simulink model "Scenario_MinimumExample_TwithTrafficLights_tol_fixed"  (R2021a)
settings: Solver=VariableStepAuto  StartTime=0.0  StopTime=50  RelTol=1e-3
model workspace (MAT data in the model file):
  Kz_dif = Simulink.Parameter
  Kz_dif.Value = Simulink.data.Expression
  Kz_dif.Value.ExpressionString = " L_dif / (Lc + ds)"
  Kz_dif.DataType = 'auto'
  Kz_dif.Dimensions = -1
  Kz_il = Simulink.Parameter
  Kz_il.Value = Simulink.data.Expression
  Kz_il.Value.ExpressionString = " L_il / (Lc + ds)"
  Kz_il.DataType = 'auto'
  Kz_il.Dimensions = -1
  Kz_ir = Simulink.Parameter
  Kz_ir.Value = Simulink.data.Expression
  Kz_ir.Value.ExpressionString = " L_ir / (Lc + ds)"
  Kz_ir.DataType = 'auto'
  Kz_ir.Dimensions = -1
  Kz_is = Simulink.Parameter
  Kz_is.Value = Simulink.data.Expression
  Kz_is.Value.ExpressionString = " L_is / (Lc + ds)"
  Kz_is.DataType = 'auto'
  Kz_is.Dimensions = -1
  Kz_long = Simulink.Parameter
  Kz_long.Value = Simulink.data.Expression
  Kz_long.Value.ExpressionString = " L_long / (Lc + ds)"
  Kz_long.Description = 'Segmentkapazität (wie viele autos passen hinein)'
  Kz_long.DataType = 'auto'
  Kz_long.Dimensions = -1
  Kz_pre = Simulink.Parameter
  Kz_pre.Value = Simulink.data.Expression
  Kz_pre.Value.ExpressionString = " L_pre / (Lc + ds)"
  Kz_pre.DataType = 'auto'
  Kz_pre.Dimensions = -1
  L_dif = Simulink.Parameter
  L_dif.Value = Simulink.data.Expression
  L_dif.Value.ExpressionString = "L_long-L_pre"
  L_dif.Description = 'Differenz zwischen Abbiegerspurlänge und normaler straßenlänge'
  L_dif.DataType = 'auto'
  L_dif.Dimensions = -1
  L_il = Simulink.Parameter
  L_il.Value = 30
  L_il.Description = 'Länge der innenkreuzungssegments, das linksabbieger durchqueren'
  L_il.DataType = 'auto'
  L_il.Dimensions = [1 1]
  L_ir = Simulink.Parameter
  L_ir.Value = 23
  L_ir.Description = 'Länge der innenkreuzungssegments, das rechtsabbieger durchqueren'
  L_ir.DataType = 'auto'
  L_ir.Dimensions = [1 1]
  L_is = Simulink.Parameter
  L_is.Value = 35
  L_is.Description = 'Länge der innenkreuzungssegments, das geradeausfahrer durchqueren'
  L_is.DataType = 'auto'
  L_is.Dimensions = [1 1]
  L_long = Simulink.Parameter
  L_long.Value = 52.8
  L_long.Description = 'Langes straßensegment  (52.8 meter)'
  L_long.DataType = 'auto'
  L_long.Dimensions = [1 1]
  L_pre = Simulink.Parameter
  L_pre.Value = 20
  L_pre.Description = 'Länge der Abbiegespuren'
  L_pre.DataType = 'auto'
  L_pre.Dimensions = [1 1]
  Lc = Simulink.Parameter
  Lc.Value = 4.4
  Lc.Description = 'Länge eines autos'
  Lc.DataType = 'auto'
  Lc.Dimensions = [1 1]
  Rk = Simulink.Parameter
  Rk.Value = Simulink.data.Expression
  Rk.Value.ExpressionString = " 1 / (Lc / v)"
  Rk.Description = 'Flussrate zwischen den Kanten (bei speed v)'
  Rk.DataType = 'auto'
  Rk.Dimensions = -1
  Tz_dif = Simulink.Parameter
  Tz_dif.Value = Simulink.data.Expression
  Tz_dif.Value.ExpressionString = " L_dif / v"
  Tz_dif.DataType = 'auto'
  Tz_dif.Dimensions = -1
  Tz_il = Simulink.Parameter
  Tz_il.Value = Simulink.data.Expression
  Tz_il.Value.ExpressionString = " L_il / v"
  Tz_il.DataType = 'auto'
  Tz_il.Dimensions = -1
  Tz_ir = Simulink.Parameter
  Tz_ir.Value = Simulink.data.Expression
  Tz_ir.Value.ExpressionString = " L_ir / v"
  Tz_ir.DataType = 'auto'
  Tz_ir.Dimensions = -1
  Tz_is = Simulink.Parameter
  Tz_is.Value = Simulink.data.Expression
  Tz_is.Value.ExpressionString = " L_is / v"
  Tz_is.DataType = 'auto'
  Tz_is.Dimensions = -1
  Tz_long = Simulink.Parameter
  Tz_long.Value = Simulink.data.Expression
  Tz_long.Value.ExpressionString = " L_long / v"
  Tz_long.Description = 'Segment durchfahrtzeit: wie lange würde ein auto brauchen,um
    | ungehindert durch das segment zu fahren.'
  Tz_long.DataType = 'auto'
  Tz_long.Dimensions = -1
  Tz_pre = Simulink.Parameter
  Tz_pre.Value = Simulink.data.Expression
  Tz_pre.Value.ExpressionString = " L_pre / v"
  Tz_pre.DataType = 'auto'
  Tz_pre.Dimensions = -1
  ds = Simulink.Parameter
  ds.Value = Simulink.data.Expression
  ds.Value.ExpressionString = "v*dt"
  ds.DataType = 'auto'
  ds.Dimensions = -1
  dt = Simulink.Parameter
  dt.Value = 1
  dt.Description = 'temporaler sicherheitsabstand'
  dt.DataType = 'auto'
  dt.Dimensions = [1 1]
  v = Simulink.Parameter
  v.Value = 13.89
  v.Description = 'geschwindigkeit eines autos
    | (km/h : 3.75 = m/s)
    | 	30km/h = 8,34m/s
    | 	20km/h = 5.56m/s
    | 	50km/h = 13.89m/s
    | '
  v.DataType = 'auto'
  v.Dimensions = [1 1]
libraries: StreetLanesLibrary x72, EdgesLibrary x64, MeasuringLibrary x33, SourcesAndSinksLibrary x12, LightsLibrary x2
(part 1 of 2)
settings Model: Creator=phill  LastModifiedBy=phill
settings SolverCC: ZeroCrossAlgorithm=Adaptive
settings DebuggingCC: IgnoredZcDiagnostic=none

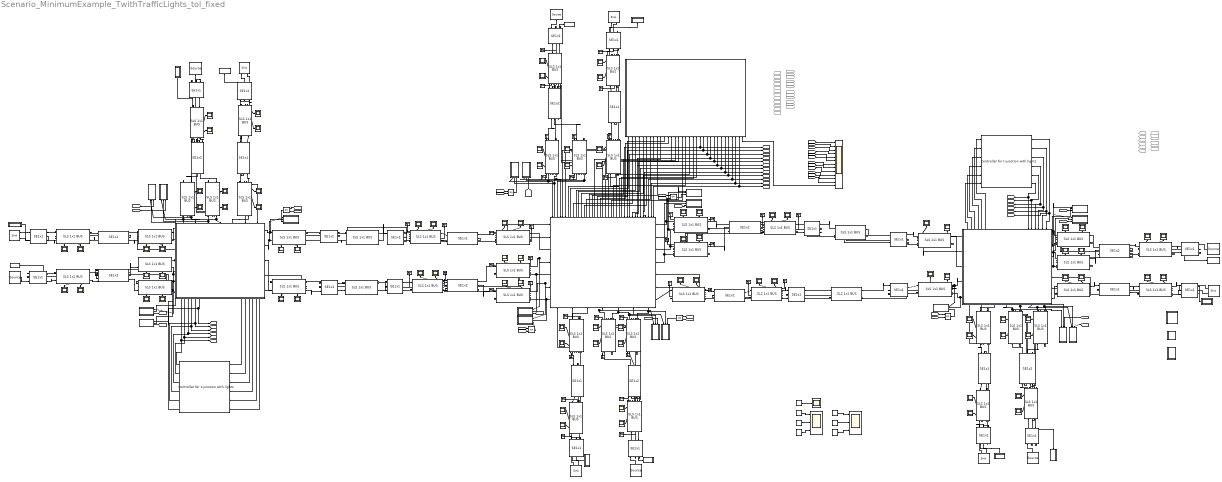
== system Scenario_MinimumExample_TwithTrafficLights_tol_fixed ==
  Ain : StreetLanesLibrary/SLS 1x1 BUS  Kz=Kz_dif  Tz=Tz_dif
  Ain2 : StreetLanesLibrary/SLS 1x1 BUS  Kz=Kz_dif  Tz=Tz_dif
  Ain3 : StreetLanesLibrary/SLS 1x1 BUS  Kz=Kz_dif  Tz=Tz_dif
  AinSplit : EdgesLibrary/SE1x2  Rk1=0.5*Rk  Rk2=0.5*Rk
  AinSplit2 : EdgesLibrary/SE1x2  Rk1=0.5*Rk  Rk2=0.5*Rk
  AinSplit3 : EdgesLibrary/SE1x2  Rk1=0.5*Rk  Rk2=0.5*Rk
  AinX : Scope
  AinX2 : Scope
  AinX3 : Scope
  AinY : Scope
  AinY2 : Scope
  AinY3 : Scope
  Al : StreetLanesLibrary/SLS 1x1 BUS  Kz=Kz_pre  Tz=Tz_pre
  AlX : Scope
  AlY : Scope
  Ali1 : StreetLanesLibrary/SLS 1x1 BUS  Kz=Kz_pre  Tz=Tz_pre
  Ali2 : StreetLanesLibrary/SLS 1x1 BUS  Kz=Kz_pre  Tz=Tz_pre
  AliX1 : Scope
  AliX2 : Scope
  AliY1 : Scope
  AliY2 : Scope
  Ao : StreetLanesLibrary/SLS 1x1 BUS  Kz=Kz_pre  Tz=Tz_pre
  Ao2 : StreetLanesLibrary/SLS 1x1 BUS  Kz=Kz_pre  Tz=Tz_pre
  Ao3 : StreetLanesLibrary/SLS 1x1 BUS  Kz=Kz_pre  Tz=Tz_pre
  AoX : Scope
  AoX2 : Scope
  AoX3 : Scope
  AoY : Scope
  AoY2 : Scope
  AoY3 : Scope
  Aout : StreetLanesLibrary/SLS 1x1 BUS  Kz=Kz_dif  Tz=Tz_dif
  Aout2 : StreetLanesLibrary/SLS 1x1 BUS  Kz=Kz_dif  Tz=Tz_dif
  Aout3 : StreetLanesLibrary/SLS 1x1 BUS  Kz=Kz_dif  Tz=Tz_dif
  AoutX : Scope
  AoutX2 : Scope
  AoutX3 : Scope
  AoutY : Scope
  AoutY2 : Scope
  AoutY3 : Scope
  Ari1 : StreetLanesLibrary/SLS 1x1 BUS  Kz=Kz_pre  Tz=Tz_pre
  Ari2 : StreetLanesLibrary/SLS 1x1 BUS  Kz=Kz_pre  Tz=Tz_pre
  AriX1 : Scope
  AriX2 : Scope
  AriY1 : Scope
  AriY2 : Scope
  Ars : StreetLanesLibrary/SLS 1x1 BUS  Kz=Kz_pre  Tz=Tz_pre
  ArsX : Scope
  ArsY : Scope
  Bin : StreetLanesLibrary/SLS 1x1 BUS  Kz=Kz_dif  Tz=Tz_dif
  BinSplit1 : EdgesLibrary/SE1x2  Rk1=0.5*Rk  Rk2=0.5*Rk
  BinX : Scope
  BinY : Scope
  Bl : StreetLanesLibrary/SLS 1x1 BUS  Kz=Kz_pre  Tz=Tz_pre
  BlX : Scope
  BlY : Scope
  Bo : StreetLanesLibrary/SLS 1x1 BUS  Kz=Kz_pre  Tz=Tz_pre
  Bo2 : StreetLanesLibrary/SLS 1x1 BUS  Kz=Kz_pre  Tz=Tz_pre
  Bo3 : StreetLanesLibrary/SLS 1x1 BUS  Kz=Kz_long  Tz=Tz_long
  Bo4 : StreetLanesLibrary/SLS 1x1 BUS  Kz=Kz_pre  Tz=Tz_pre
  BoX : Scope
  BoX2 : Scope
  BoX3 : Scope
  BoY : Scope
  BoY2 : Scope
  BoY3 : Scope
  Bout : StreetLanesLibrary/SLS 1x1 BUS  Kz=Kz_dif  Tz=Tz_dif
  BoutX : Scope
  BoutY : Scope
  Brs : StreetLanesLibrary/SLS 1x1 BUS  Kz=Kz_pre  Tz=Tz_pre
  Brs2 : StreetLanesLibrary/SLS 1x1 BUS  Kz=Kz_pre  Tz=Tz_pre
  Brs3 : StreetLanesLibrary/SLS 1x1 BUS  Kz=Kz_long  Tz=Tz_long
  Brs4 : StreetLanesLibrary/SLS 1x1 BUS  Kz=Kz_pre  Tz=Tz_pre
  BrsX : Scope
  BrsX2 : Scope
  BrsX3 : Scope
  BrsY : Scope
  BrsY2 : Scope
  BrsY3 : Scope
  Cin : StreetLanesLibrary/SLS 1x1 BUS  Kz=Kz_dif  Tz=Tz_dif
  Cin2 : StreetLanesLibrary/SLS 1x1 BUS  Kz=Kz_dif  Tz=Tz_dif
  Cin3 : StreetLanesLibrary/SLS 1x1 BUS  Kz=Kz_long  Tz=Tz_long
  Cin4 : StreetLanesLibrary/SLS 1x1 BUS  Kz=Kz_dif  Tz=Tz_dif
  CinSplit : EdgesLibrary/SE1x2  Rk1=0.5*Rk  Rk2=0.5*Rk
  CinSplit2 : EdgesLibrary/SE1x2  Rk1=0.5*Rk  Rk2=0.5*Rk
  CinSplit3 : EdgesLibrary/SE1x2  Rk1=0.5*Rk  Rk2=0.5*Rk
  CinX : Scope
  CinX2 : Scope
  CinX3 : Scope
  CinY : Scope
  CinY2 : Scope
  CinY3 : Scope
  Cl : StreetLanesLibrary/SLS 1x1 BUS  Kz=Kz_pre  Tz=Tz_pre
  Cl2 : StreetLanesLibrary/SLS 1x1 BUS  Kz=Kz_pre  Tz=Tz_pre
  Cl3 : StreetLanesLibrary/SLS 1x1 BUS  Kz=Kz_pre  Tz=Tz_pre
  ClX : Scope
  ClX2 : Scope
  ClX3 : Scope
  ClY1 : Scope
  ClY2 : Scope
  Cly : Scope
  Co : StreetLanesLibrary/SLS 1x1 BUS  Kz=Kz_pre  Tz=Tz_pre
  Co2 : StreetLanesLibrary/SLS 1x1 BUS  Kz=Kz_pre  Tz=Tz_pre
  Co3 : StreetLanesLibrary/SLS 1x1 BUS  Kz=Kz_pre  Tz=Tz_pre
  CoX : Scope
  CoX2 : Scope
  CoX3 : Scope
  CoY : Scope
  CoY2 : Scope
  CoY3 : Scope
  Controller for t-junction with lights : LightsLibrary/Controller for t-junction with lights  green_time=5
  Controller for t-junction with lights1 : LightsLibrary/Controller for t-junction with lights  green_time=5
  Cout{,2..4} (4 alike) : StreetLanesLibrary/SLS 1x1 BUS  Kz=Kz_dif  Tz=Tz_dif
  CoutX : Scope
  CoutX2 : Scope
  CoutX3 : Scope
  CoutY : Scope
  CoutY2 : Scope
  CoutY3 : Scope
  Crs : StreetLanesLibrary/SLS 1x1 BUS  Kz=Kz_pre  Tz=Tz_pre
  CrsX : Scope
  CrsY : Scope
  Cs1 : StreetLanesLibrary/SLS 1x1 BUS  Kz=Kz_pre  Tz=Tz_pre
  Cs2 : StreetLanesLibrary/SLS 1x1 BUS  Kz=Kz_pre  Tz=Tz_pre
  CsX1 : Scope
  CsX2 : Scope
  CsY1 : Scope
  CsY2 : Scope
  Din : StreetLanesLibrary/SLS 1x1 BUS  Kz=Kz_dif  Tz=Tz_dif
  DinSplit : EdgesLibrary/SE1x2  Rk1=0.5*Rk  Rk2=0.5*Rk
  DinX : Scope
  DinY : Scope
  Dl : StreetLanesLibrary/SLS 1x1 BUS  Kz=Kz_pre  Tz=Tz_pre
  DlX : Scope
  DlY : Scope
  Do : StreetLanesLibrary/SLS 1x1 BUS  Kz=Kz_pre  Tz=Tz_pre
  DoX : Scope
  DoY : Scope
  Dout : StreetLanesLibrary/SLS 1x1 BUS  Kz=Kz_dif  Tz=Tz_dif
  DoutX : Scope
  DoutY : Scope
  Drs : StreetLanesLibrary/SLS 1x1 BUS  Kz=Kz_pre  Tz=Tz_pre
  DrsX : Scope
  DrsY : Scope
  From24 : From  Commented=on  GotoTag=CenAl
  From25 : From  Commented=on  GotoTag=CenAs
  From26 : From  Commented=on  GotoTag=CenDs
  From27 : From  Commented=on  GotoTag=CenDr
  From28 : From  Commented=on  GotoTag=CenAr
  From29 : From  Commented=on  GotoTag=CenBl
  From30 : From  Commented=on  GotoTag=CenBs
  From31 : From  Commented=on  GotoTag=CenBr
  From32 : From  Commented=on  GotoTag=CenCl
  From33 : From  Commented=on  GotoTag=CenCs
  From34 : From  Commented=on  GotoTag=CenCr
  From35 : From  Commented=on  GotoTag=CenDl
  From42 : From  Commented=on  GotoTag=RenCs
  From43 : From  Commented=on  GotoTag=RenCl
  From44 : From  Commented=on  GotoTag=RenAr
  From45 : From  Commented=on  GotoTag=RenAl
  From46 : From  Commented=on  GotoTag=RenBr
  From47 : From  Commented=on  GotoTag=RenBs
  Goto24 : Goto  Commented=on  GotoTag=CenAl
  Goto25 : Goto  Commented=on  GotoTag=CenAs
  Goto26 : Goto  Commented=on  GotoTag=CenDs
  Goto27 : Goto  Commented=on  GotoTag=CenDr
  Goto28 : Goto  Commented=on  GotoTag=CenAr
  Goto29 : Goto  Commented=on  GotoTag=CenBl
  Goto30 : Goto  Commented=on  GotoTag=CenBs
  Goto31 : Goto  Commented=on  GotoTag=CenBr
  Goto32 : Goto  Commented=on  GotoTag=CenCl
  Goto33 : Goto  Commented=on  GotoTag=CenCs
  Goto34 : Goto  Commented=on  GotoTag=CenCr
  Goto35 : Goto  Commented=on  GotoTag=CenDl
  Goto42 : Goto  Commented=on  GotoTag=RenCl
  Goto43 : Goto  Commented=on  GotoTag=RenCs
  Goto44 : Goto  Commented=on  GotoTag=RenBs
  Goto45 : Goto  Commented=on  GotoTag=RenBr
  Goto46 : Goto  Commented=on  GotoTag=RenAl
  Goto47 : Goto  Commented=on  GotoTag=RenAr
  Kz_dif : Constant  Value=Kz_dif
  Kz_long : Constant  Value=Kz_long
  Kz_pre : Constant  Value=Kz_pre
  Kzs : Scope  NumInputPorts=3
  Logical Operator{,1..5} (6 alike) : Logic  Operator=OR  AllPortsSameDT=off  OutDataTypeStr=boolean
  Plus-Controller : Stateflow chart  TreatAsAtomicUnit=on  mask{green_duration_sr=6, green_duration_l=6, tol=0}
      mask prompts: green_duration_sr "Green Duration for straight/right traffic"; green_duration_l "Green Duration for left traffic"; tol "tolerance"
      settings: PortSchema="{\"entries\":[{\"content\":{\"sides\":[{\"content\":{\"connectorIds\":[]},\"type\":\"ConnectorPlacement.EquallySpacedRectSide\",\"uuid\":\"2590cc03-86a2-4387-8b1b-fdf4c8b68aa6\"},{\"content\":{\"connectorIds\":[],\"side\":\"RIGHT\"},\"type\":\"ConnectorPlacement.EquallySpacedRectSide\",\"uuid\":\"b97063cd-dd31-425f-b4aa-3aaa013ac411\"},{\"content\":{\"connectorIds\":[],\"side\":\"TOP\"},\"type\":\"ConnectorPlacement.EquallySpacedRectSide\",\"uuid\":\"ef5846b9-436e-4b10-a854-1305521b6a0d\"},{\"content\":{\"connectorIds\":[\"In3\",\"In4\",\"In1\",\"In2\",\"In5\",\"In6\",\"In7\",\"In8\",\"In9\",\"In10\",\"In11\",\"In12\",\"In13\",\"In14\",\"In15\",\"In16\",\"In17\",\"In18\",\"In19\",\"In20\",\"Out1\",\"Out2\",\"Out3\",\"Out4\",\"Out5\",\"Out6\",\"Out7\",\"Out8\",\"Out9\",\"Out10\",\"Out11\",\"Out12\",\"Out13\"],\"side\":\"BOTTOM\"},\"type\":\"ConnectorPlacement.EquallySpacedRectSide\",\"uuid\":\"44b73820-3b7c-4ee5-b5da-9465e85a924e\"}]},\"type\":\"ConnectorPlacement.EquallySpacedConnector\",\"uuid\":\"3342797d-7762-4a2a-891a-654024402a66\"}],\"packageUris\":[\"http://schema.mathworks.com/mf0/Connector/R2020b\"],\"version\":\"1.0\"}"
  Rk : Constant  Value=Rk
  SE1x{1..4,7..10} (8 alike) : EdgesLibrary/SE1x1  Rk=Rk  slope=2000
  Scope : Scope  NumInputPorts=13
  Sink A : SourcesAndSinksLibrary/Sink  SystemSampleTime=-1  VariantActivationTime=update diagram  Latency=0  AutoFrameSizeCalculation=off
      settings: PortSchema="{\"entries\":[{\"content\":{\"sides\":[{\"content\":{\"connectorIds\":[\"Out1\",\"Out2\"]},\"type\":\"ConnectorPlacement.EquallySpacedRectSide\",\"uuid\":\"9fd2383e-3590-4f0f-bafc-5a4adfbb32b4\"},{\"content\":{\"connectorIds\":[],\"side\":\"RIGHT\"},\"type\":\"ConnectorPlacement.EquallySpacedRectSide\",\"uuid\":\"1e687aa9-1098-45bd-a1f6-ea403f3f2897\"},{\"content\":{\"connectorIds\":[],\"side\":\"TOP\"},\"type\":\"ConnectorPlacement.EquallySpacedRectSide\",\"uuid\":\"fe6eaa71-085c-414b-983a-a0e72e52a49c\"}]},\"type\":\"ConnectorPlacement.EquallySpacedConnector\",\"uuid\":\"370c1712-4373-4726-99c2-6cb04807ece1\"}],\"packageUris\":[\"http://schema.mathworks.com/mf0/Connector/R2020b\"],\"version\":\"1.0\"}"
  Sink A2 : SourcesAndSinksLibrary/Sink  SystemSampleTime=-1  VariantActivationTime=update diagram  Latency=0  AutoFrameSizeCalculation=off
      settings: PortSchema="{\"entries\":[{\"content\":{\"sides\":[{\"content\":{\"connectorIds\":[\"Out1\",\"Out2\"]},\"type\":\"ConnectorPlacement.EquallySpacedRectSide\",\"uuid\":\"9fd2383e-3590-4f0f-bafc-5a4adfbb32b4\"},{\"content\":{\"connectorIds\":[],\"side\":\"RIGHT\"},\"type\":\"ConnectorPlacement.EquallySpacedRectSide\",\"uuid\":\"1e687aa9-1098-45bd-a1f6-ea403f3f2897\"},{\"content\":{\"connectorIds\":[],\"side\":\"TOP\"},\"type\":\"ConnectorPlacement.EquallySpacedRectSide\",\"uuid\":\"fe6eaa71-085c-414b-983a-a0e72e52a49c\"}]},\"type\":\"ConnectorPlacement.EquallySpacedConnector\",\"uuid\":\"370c1712-4373-4726-99c2-6cb04807ece1\"}],\"packageUris\":[\"http://schema.mathworks.com/mf0/Connector/R2020b\"],\"version\":\"1.0\"}"
  Sink A3 : SourcesAndSinksLibrary/Sink  SystemSampleTime=-1  VariantActivationTime=update diagram  Latency=0  AutoFrameSizeCalculation=off
      settings: PortSchema="{\"entries\":[{\"content\":{\"sides\":[{\"content\":{\"connectorIds\":[\"Out1\",\"Out2\"]},\"type\":\"ConnectorPlacement.EquallySpacedRectSide\",\"uuid\":\"9fd2383e-3590-4f0f-bafc-5a4adfbb32b4\"},{\"content\":{\"connectorIds\":[],\"side\":\"RIGHT\"},\"type\":\"ConnectorPlacement.EquallySpacedRectSide\",\"uuid\":\"1e687aa9-1098-45bd-a1f6-ea403f3f2897\"},{\"content\":{\"connectorIds\":[],\"side\":\"TOP\"},\"type\":\"ConnectorPlacement.EquallySpacedRectSide\",\"uuid\":\"fe6eaa71-085c-414b-983a-a0e72e52a49c\"}]},\"type\":\"ConnectorPlacement.EquallySpacedConnector\",\"uuid\":\"370c1712-4373-4726-99c2-6cb04807ece1\"}],\"packageUris\":[\"http://schema.mathworks.com/mf0/Connector/R2020b\"],\"version\":\"1.0\"}"
  Sink C : SourcesAndSinksLibrary/Sink  SystemSampleTime=-1  VariantActivationTime=update diagram  Latency=0  AutoFrameSizeCalculation=off
      settings: PortSchema="{\"entries\":[{\"content\":{\"sides\":[{\"content\":{\"connectorIds\":[\"Out1\",\"Out2\"]},\"type\":\"ConnectorPlacement.EquallySpacedRectSide\",\"uuid\":\"9fd2383e-3590-4f0f-bafc-5a4adfbb32b4\"},{\"content\":{\"connectorIds\":[],\"side\":\"RIGHT\"},\"type\":\"ConnectorPlacement.EquallySpacedRectSide\",\"uuid\":\"1e687aa9-1098-45bd-a1f6-ea403f3f2897\"},{\"content\":{\"connectorIds\":[],\"side\":\"TOP\"},\"type\":\"ConnectorPlacement.EquallySpacedRectSide\",\"uuid\":\"fe6eaa71-085c-414b-983a-a0e72e52a49c\"}]},\"type\":\"ConnectorPlacement.EquallySpacedConnector\",\"uuid\":\"370c1712-4373-4726-99c2-6cb04807ece1\"}],\"packageUris\":[\"http://schema.mathworks.com/mf0/Connector/R2020b\"],\"version\":\"1.0\"}"
  Sink C2 : SourcesAndSinksLibrary/Sink  SystemSampleTime=-1  VariantActivationTime=update diagram  Latency=0  AutoFrameSizeCalculation=off
      settings: PortSchema="{\"entries\":[{\"content\":{\"sides\":[{\"content\":{\"connectorIds\":[\"Out1\",\"Out2\"]},\"type\":\"ConnectorPlacement.EquallySpacedRectSide\",\"uuid\":\"9fd2383e-3590-4f0f-bafc-5a4adfbb32b4\"},{\"content\":{\"connectorIds\":[],\"side\":\"RIGHT\"},\"type\":\"ConnectorPlacement.EquallySpacedRectSide\",\"uuid\":\"1e687aa9-1098-45bd-a1f6-ea403f3f2897\"},{\"content\":{\"connectorIds\":[],\"side\":\"TOP\"},\"type\":\"ConnectorPlacement.EquallySpacedRectSide\",\"uuid\":\"fe6eaa71-085c-414b-983a-a0e72e52a49c\"}]},\"type\":\"ConnectorPlacement.EquallySpacedConnector\",\"uuid\":\"370c1712-4373-4726-99c2-6cb04807ece1\"}],\"packageUris\":[\"http://schema.mathworks.com/mf0/Connector/R2020b\"],\"version\":\"1.0\"}"
  Sink D : SourcesAndSinksLibrary/Sink  SystemSampleTime=-1  VariantActivationTime=update diagram  Latency=0  AutoFrameSizeCalculation=off
      settings: PortSchema="{\"entries\":[{\"content\":{\"sides\":[{\"content\":{\"connectorIds\":[\"Out1\",\"Out2\"]},\"type\":\"ConnectorPlacement.EquallySpacedRectSide\",\"uuid\":\"9fd2383e-3590-4f0f-bafc-5a4adfbb32b4\"},{\"content\":{\"connectorIds\":[],\"side\":\"RIGHT\"},\"type\":\"ConnectorPlacement.EquallySpacedRectSide\",\"uuid\":\"1e687aa9-1098-45bd-a1f6-ea403f3f2897\"},{\"content\":{\"connectorIds\":[],\"side\":\"TOP\"},\"type\":\"ConnectorPlacement.EquallySpacedRectSide\",\"uuid\":\"fe6eaa71-085c-414b-983a-a0e72e52a49c\"}]},\"type\":\"ConnectorPlacement.EquallySpacedConnector\",\"uuid\":\"370c1712-4373-4726-99c2-6cb04807ece1\"}],\"packageUris\":[\"http://schema.mathworks.com/mf0/Connector/R2020b\"],\"version\":\"1.0\"}"
  Source A : SourcesAndSinksLibrary/Source  SystemSampleTime=-1  VariantActivationTime=update diagram  Latency=0  AutoFrameSizeCalculation=off
  Source A2 : SourcesAndSinksLibrary/Source  SystemSampleTime=-1  VariantActivationTime=update diagram  Latency=0  AutoFrameSizeCalculation=off
  Source A3 : SourcesAndSinksLibrary/Source  SystemSampleTime=-1  VariantActivationTime=update diagram  Latency=0  AutoFrameSizeCalculation=off
  Source C : SourcesAndSinksLibrary/Source  SystemSampleTime=-1  VariantActivationTime=update diagram  Latency=0  AutoFrameSizeCalculation=off
  Source C2 : SourcesAndSinksLibrary/Source  SystemSampleTime=-1  VariantActivationTime=update diagram  Latency=0  AutoFrameSizeCalculation=off
  Source D : SourcesAndSinksLibrary/Source  SystemSampleTime=-1  VariantActivationTime=update diagram  Latency=0  AutoFrameSizeCalculation=off
  Subsystem : Subsystem  mask{Kz_left=Kz_il, Tz_left=Tz_il, Kz_straight=Kz_is, Tz_straight=Tz_is, Kz_right=Kz_ir, Tz_right=Tz_ir, Rk=Rk}
      settings: PortSchema="{\"entries\":[{\"content\":{\"sides\":[{\"content\":{\"connectorIds\":[\"In1\",\"In2\",\"Out30\",\"In3\",\"Out31\",\"In4\",\"Out32\"]},\"type\":\"ConnectorPlacement.EquallySpacedRectSide\",\"uuid\":\"223afcc5-5490-41e2-b2c1-0ac31bdd31f0\"},{\"content\":{\"connectorIds\":[\"In25\",\"Out1\",\"In26\",\"Out2\",\"In27\",\"In28\",\"Out3\"],\"side\":\"RIGHT\"},\"type\":\"ConnectorPlacement.EquallySpacedRectSide\",\"uuid\":\"e803e5ea-345a-49fc-8782-ffb100729ba0\"},{\"content\":{\"connectorIds\":[\"In5\",\"Out7\",\"Out8\",\"In6\",\"In7\",\"In8\",\"Out9\",\"Out10\",\"Out11\",\"Out12\",\"Out13\",\"Out14\",\"Out15\",\"Out16\",\"Out17\",\"Out18\",\"Out19\",\"Out20\",\"Out21\",\"Out22\",\"Out23\",\"Out24\",\"Out25\",\"Out26\",\"Out27\",\"Out28\",\"Out29\",\"In9\",\"In10\",\"In11\",\"In12\",\"In13\",\"In14\",\"In15\",\"In16\",\"In17\",\"In18\",\"In19\",\"In20\"],\"side\":\"TOP\"},\"type\":\"ConnectorPlacement.EquallySpacedRectSide\",\"uuid\":\"8581fbf9-6742-4a7a-9e93-ed29b1a56c31\"},{\"content\":{\"connectorIds\":[\"In21\",\"In22\",\"Out4\",\"In23\",\"Out5\",\"In24\",\"Out6\"],\"side\":\"BOTTOM\"},\"type\":\"ConnectorPlacement.EquallySpacedRectSide\",\"uuid\":\"cc67de78-9dd9-463d-9445-caa2eb7c099b\"}]},\"type\":\"ConnectorPlacement.EquallySpacedConnector\",\"uuid\":\"ac6fc4cc-2326-4bcf-896c-a5d089a8f47a\"}],\"packageUris\":[\"http://schema.mathworks.com/mf0/Connector/R2020b\"],\"version\":\"1.0\"}"
      mask Display:
      | %image('$imagefile'); % Use "Edit Image" on toolstrip to change.
      | disp('+ \n\n');
      | KzS = get_param(gcb,'Kz_straight');
      | TzS = get_param(gcb,'Tz_straight');
      | KzR = get_param(gcb,'Kz_right');
      | TzR = get_param(gcb,'Tz_right');
      | KzL = get_param(gcb,'Kz_left');
      | TzL = get_param(gcb,'Tz_left');
      | Rk = get_param(gcb,'Rk');
      | disp(['Rk = ', Rk, ' | Kz/Tz L = ', KzL, ' ', TzL, ' | Kz/Tz S = ', KzS, ' ', TzS, ' | Kz/Tz R = ', KzR, ' ', TzR]);
  Subsystem1 : Subsystem  mask{Kz_left=Kz_il, Tz_left=Tz_il, Kz_straight=Kz_is, Tz_straight=Tz_is, Kz_right=Kz_ir, Tz_right=Tz_ir, Rk=Rk}
      settings: PortSchema="{\"entries\":[{\"content\":{\"sides\":[{\"content\":{\"connectorIds\":[\"In1\",\"In2\",\"Out24\",\"In3\",\"Out25\"]},\"type\":\"ConnectorPlacement.EquallySpacedRectSide\",\"uuid\":\"96c9f498-b0bc-4839-a476-8992d885d35a\"},{\"content\":{\"connectorIds\":[\"In14\",\"Out1\",\"In15\",\"Out2\",\"In16\",\"In17\",\"Out3\"],\"side\":\"RIGHT\"},\"type\":\"ConnectorPlacement.EquallySpacedRectSide\",\"uuid\":\"11ab0cdd-7db6-4f39-a252-8216aa6322d2\"},{\"content\":{\"connectorIds\":[\"Out7\",\"Out8\",\"Out9\",\"Out10\",\"Out11\",\"Out12\",\"Out13\",\"Out14\",\"Out15\",\"Out16\",\"Out17\",\"Out18\",\"Out19\",\"Out20\",\"Out21\",\"Out22\",\"Out23\",\"In4\",\"In5\",\"In6\",\"In7\",\"In8\",\"In9\"],\"side\":\"TOP\"},\"type\":\"ConnectorPlacement.EquallySpacedRectSide\",\"uuid\":\"f8ff7b80-df82-4633-b83a-80e44c4409b9\"},{\"content\":{\"connectorIds\":[\"In10\",\"In11\",\"Out4\",\"In12\",\"Out5\",\"In13\",\"Out6\"],\"side\":\"BOTTOM\"},\"type\":\"ConnectorPlacement.EquallySpacedRectSide\",\"uuid\":\"816219a6-152c-447e-807e-ad4d62c96b47\"}]},\"type\":\"ConnectorPlacement.EquallySpacedConnector\",\"uuid\":\"16c591aa-9a6b-4cb9-9c60-a78ca06e8a6b\"}],\"packageUris\":[\"http://schema.mathworks.com/mf0/Connector/R2020b\"],\"version\":\"1.0\"}"
      mask Display:
      | %image('$imagefile'); % Use "Edit Image" on toolstrip to change.
      | disp('T \n\n');
      | KzS = get_param(gcb,'Kz_straight');
      | TzS = get_param(gcb,'Tz_straight');
      | KzR = get_param(gcb,'Kz_right');
      | TzR = get_param(gcb,'Tz_right');
      | KzL = get_param(gcb,'Kz_left');
      | TzL = get_param(gcb,'Tz_left');
      | Rk = get_param(gcb,'Rk');
      | disp(['Rk = ', Rk, ' | Kz/Tz L = ', KzL, ' ', TzL, ' | Kz/Tz S = ', KzS, ' ', TzS, ' | Kz/Tz R = ', KzR, ' ', TzR]);
  Subsystem3 : Subsystem  mask{Kz_left=Kz_il, Tz_left=Tz_il, Kz_straight=Kz_is, Tz_straight=Tz_is, Kz_right=Kz_ir, Tz_right=Tz_ir, Rk=Rk}
      settings: PortSchema="{\"entries\":[{\"content\":{\"sides\":[{\"content\":{\"connectorIds\":[\"In1\",\"In2\",\"Out24\",\"In3\",\"Out25\"]},\"type\":\"ConnectorPlacement.EquallySpacedRectSide\",\"uuid\":\"96c9f498-b0bc-4839-a476-8992d885d35a\"},{\"content\":{\"connectorIds\":[\"In14\",\"Out1\",\"In15\",\"Out2\",\"In16\",\"In17\",\"Out3\"],\"side\":\"RIGHT\"},\"type\":\"ConnectorPlacement.EquallySpacedRectSide\",\"uuid\":\"11ab0cdd-7db6-4f39-a252-8216aa6322d2\"},{\"content\":{\"connectorIds\":[\"Out7\",\"Out8\",\"Out9\",\"Out10\",\"Out11\",\"Out12\",\"Out13\",\"Out14\",\"Out15\",\"Out16\",\"Out17\",\"Out18\",\"Out19\",\"Out20\",\"Out21\",\"Out22\",\"Out23\",\"In4\",\"In5\",\"In6\",\"In7\",\"In8\",\"In9\"],\"side\":\"TOP\"},\"type\":\"ConnectorPlacement.EquallySpacedRectSide\",\"uuid\":\"f8ff7b80-df82-4633-b83a-80e44c4409b9\"},{\"content\":{\"connectorIds\":[\"In10\",\"In11\",\"Out4\",\"In12\",\"Out5\",\"In13\",\"Out6\"],\"side\":\"BOTTOM\"},\"type\":\"ConnectorPlacement.EquallySpacedRectSide\",\"uuid\":\"816219a6-152c-447e-807e-ad4d62c96b47\"}]},\"type\":\"ConnectorPlacement.EquallySpacedConnector\",\"uuid\":\"16c591aa-9a6b-4cb9-9c60-a78ca06e8a6b\"}],\"packageUris\":[\"http://schema.mathworks.com/mf0/Connector/R2020b\"],\"version\":\"1.0\"}"
      mask Display:
      | %image('$imagefile'); % Use "Edit Image" on toolstrip to change.
      | disp('T \n\n');
      | KzS = get_param(gcb,'Kz_straight');
      | TzS = get_param(gcb,'Tz_straight');
      | KzR = get_param(gcb,'Kz_right');
      | TzR = get_param(gcb,'Tz_right');
      | KzL = get_param(gcb,'Kz_left');
      | TzL = get_param(gcb,'Tz_left');
      | Rk = get_param(gcb,'Rk');
      | disp(['Rk = ', Rk, ' | Kz/Tz L = ', KzL, ' ', TzL, ' | Kz/Tz S = ', KzS, ' ', TzS, ' | Kz/Tz R = ', KzR, ' ', TzR]);
  Terminator{1..7,10..16,19..25,28..34,37..48} (40 alike) : Terminator
  Tz_dif : Constant  Value=Tz_dif
  Tz_long : Constant  Value=Tz_long
  Tz_pre : Constant  Value=Tz_pre
  Tzs : Scope  NumInputPorts=3
  Tzs1 : Scope
  deadtimes : Subsystem
  deadtimes1 : Subsystem
  deadtimes10 : Subsystem
  deadtimes11 : Subsystem
  deadtimes12 : Subsystem
  deadtimes13 : Subsystem
  deadtimes14 : Subsystem
  deadtimes15 : Subsystem
  deadtimes16 : Subsystem
  deadtimes17 : Subsystem
  deadtimes2 : Subsystem
  deadtimes3 : Subsystem
  deadtimes4 : Subsystem
  deadtimes5 : Subsystem
  deadtimes6 : Subsystem
  deadtimes7 : Subsystem
  deadtimes8 : Subsystem
  deadtimes9 : Subsystem
  from Source A : EdgesLibrary/SE1x1  Rk=Rk  slope=2000
  from Source A2 : EdgesLibrary/SE1x1  Rk=Rk  slope=2000
  from Source A3 : EdgesLibrary/SE1x1  Rk=Rk  slope=2000
  from Source B : EdgesLibrary/SE1x1  Rk=Rk  slope=2000
  from Source B2 : EdgesLibrary/SE1x1  Rk=Rk  slope=2000
  from Source B3 : EdgesLibrary/SE1x1  Rk=Rk  slope=2000
  from Source C : EdgesLibrary/SE1x1  Rk=Rk  slope=2000
  from Source C2 : EdgesLibrary/SE1x1  Rk=Rk  slope=2000
  from Source C3 : EdgesLibrary/SE1x1  Rk=Rk  slope=2000
  from Source D : EdgesLibrary/SE1x1  Rk=Rk  slope=2000
  rel xz : Subsystem  AncestorBlock=MeasuringLibrary/rel xz scope
  sinks : Subsystem  AncestorBlock=MeasuringLibrary/sink_edge_checker_scope  mask{shortestPathTz=0}
      mask prompts: shortestPathTz "Sum of Tz on the path to the closest source"
      mask Display: disp(['pathTz = ', get_param(gcb,'shortestPathTz')])
  sinks1 : Subsystem  mask{shortestPathTz=2*Tz_dif+2*Tz_pre+Tz_ir}
      mask prompts: shortestPathTz "Sum of Tz on the path to the closest source"
      mask Display: disp(['pathTz = ', get_param(gcb,'shortestPathTz')])
  sinks2 : Subsystem  mask{shortestPathTz=2*Tz_dif+2*Tz_pre+Tz_il}
      mask prompts: shortestPathTz "Sum of Tz on the path to the closest source"
      mask Display: disp(['pathTz = ', get_param(gcb,'shortestPathTz')])
  sinks3 : Subsystem  mask{shortestPathTz=2*Tz_dif+2*Tz_pre+Tz_is}
      mask prompts: shortestPathTz "Sum of Tz on the path to the closest source"
      mask Display: disp(['pathTz = ', get_param(gcb,'shortestPathTz')])
  sinks4 : Subsystem  mask{shortestPathTz=2*Tz_dif+2*Tz_pre+Tz_is}
      mask prompts: shortestPathTz "Sum of Tz on the path to the closest source"
      mask Display: disp(['pathTz = ', get_param(gcb,'shortestPathTz')])
  sinks5 : Subsystem  mask{shortestPathTz=2*Tz_dif+2*Tz_pre+Tz_il}
      mask prompts: shortestPathTz "Sum of Tz on the path to the closest source"
      mask Display: disp(['pathTz = ', get_param(gcb,'shortestPathTz')])
  sinks6 : Subsystem  mask{shortestPathTz=2*Tz_dif+2*Tz_pre+Tz_ir}
      mask prompts: shortestPathTz "Sum of Tz on the path to the closest source"
      mask Display: disp(['pathTz = ', get_param(gcb,'shortestPathTz')])
  sources : Subsystem  AncestorBlock=MeasuringLibrary/source_edge_checker_scope
  sources1 : Subsystem
  sources2 : Subsystem
  sources4 : Subsystem
  sources5 : Subsystem
  sources6 : Subsystem
  sources7 : MeasuringLibrary/source_edge_checker_scope  SystemSampleTime=-1  VariantActivationTime=update diagram  Latency=0  AutoFrameSizeCalculation=off
  to Sink A : EdgesLibrary/SE1x1  Rk=Rk  slope=2000
  to Sink A2 : EdgesLibrary/SE1x1  Rk=Rk  slope=2000
  to Sink A3 : EdgesLibrary/SE1x1  Rk=Rk  slope=2000
  to Sink B : EdgesLibrary/SE1x1  Rk=Rk  slope=2000
  to Sink B2 : EdgesLibrary/SE1x1  Rk=Rk  slope=2000
  to Sink B3 : EdgesLibrary/SE1x1  Rk=Rk  slope=2000
  to Sink C : EdgesLibrary/SE1x1  Rk=Rk  slope=2000
  to Sink C2 : EdgesLibrary/SE1x1  Rk=Rk  slope=2000
  to Sink C3 : EdgesLibrary/SE1x1  Rk=Rk  slope=2000
  to Sink D : EdgesLibrary/SE1x1  Rk=Rk  slope=2000
  wires:
  Cout3/2 -> from Source B3/1
  Brs3/2 -> from Source B2/1
  Sink A/1 -> to Sink A/2
  Ao/3 -> AoX/1
  Kz_long/1 -> Kzs/1  "Kz_long"
  Ain/4 -> AinY/1
  Ain/3 -> AinX/1
  Bo/2 -> SE1x2/1
  Ain/6 -> from Source A/2
  Al/3 -> AlX/1
  Bl/4 -> BlY/1
  from Source A/1 -> Ain/1
  Source A/1 -> from Source A/1
  Aout/3 -> AoutX/1
  Aout/6 -> SE1x1/2
  Bl/3 -> BlX/1
  Cin/7 -> from Source C/3
  to Sink A/2 -> Aout/2
  Aout/4 -> AoutY/1
  Aout/7 -> SE1x1/3
  Ain/2 -> AinSplit/1
  Bl/7 -> BinSplit1/3
  DinSplit/2 -> Dl/1
  Ao/5 -> Terminator2/1
  Cin/3 -> CinX/1
  Din/5 -> Terminator34/1
  Subsystem/9(Do yk) -> Do/1
  Dl/1 -> Terminator30/1
  Ars/6 -> AinSplit/4
  Al/6 -> AinSplit/2
  Ain/5 -> Terminator7/1
  Bo/4 -> BoY/1
  Co/6 -> Subsystem/27(Co x)
  Cout/4 -> CoutY/1
  Cl/1 -> Terminator22/1
  Brs/5 -> Terminator48/1
  Bout/7 -> SE1x2/3
  Co/4 -> CoY/1
  Co/5 -> Terminator20/1
  Crs/4 -> CrsY/1
  SE1x2/1 -> Bout/1
  CinSplit/3 -> Cin/2
  Cl/6 -> CinSplit/4
  Ao/4 -> AoY/1
  Cout/5 -> Terminator23/1
  Din/6 -> from Source D/2
  Drs/1 -> Terminator31/1
  SE1x3/1 -> Cout/1
  Crs/6 -> CinSplit/2
  from Source C/1 -> Cin/1
  Cout/7 -> SE1x3/3
  Cin/6 -> from Source C/2
  Tz_pre/1 -> Tzs/2  "Tz_pre"
  Brs/3 -> BrsX/1
  Do/4 -> DoY/1
  to Sink D/2 -> Dout/2
  Ars/4 -> ArsY/1
  Din/4 -> DinY/1
  to Sink C/2 -> Cout/2
  to Sink D/1 -> sinks4/1(edge)
  Aout/2 -> to Sink A/1
  Ain/7 -> from Source A/3
  Drs/3 -> DrsX/1
  Dout/3 -> DoutX/1
  Source D/1 -> from Source D/1
  Ars/7 -> AinSplit/5
  Dl/4 -> DlY/1
  Bin/3 -> BinX/1
  Dout/4 -> DoutY/1
  Dl/5 -> Terminator43/1
  DinSplit/1 -> Drs/1
  Bin/7 -> from Source B/3
  from Source D/2 -> sources5/1(edge)
  Dl/6 -> DinSplit/4
  Din/2 -> DinSplit/1
  Cl/7 -> CinSplit/5
  Sink D/2 -> to Sink D/3
  Ao/2 -> SE1x1/1
  Do/2 -> SE1x4/1
  SE1x2/2 -> Bo/2
  Din/1 -> Terminator28/1
  Ari1/4 -> AriY1/1
  Dl/3 -> DlX/1
  Co/1 -> Terminator39/1
  Bo/7 -> Subsystem/2(Bo Kz)
  Tz_long/1 -> Tzs/1  "Tz_long"
  Do/5 -> Terminator29/1
  Do/3 -> DoX/1
  Kz_dif/1 -> Kzs/3  "Kz_dif"
  BinSplit1/1 -> Bl/1
  Ars/3 -> ArsX/1
  Cin/1 -> Terminator19/1
  AinSplit/2 -> Ars/1
  Bout/1 -> Terminator15/1
  Co/3 -> CoX/1
  Crs/1 -> Terminator21/1
  SE1x1/1 -> Aout/1
  Crs/7 -> CinSplit/3
  Crs/5 -> Terminator37/1
  Al/4 -> AlY/1
  Cout/3 -> CoutX/1
  Co/7 -> Subsystem/28(Co Kz)
  Bout/5 -> Terminator14/1
  Bout/2 -> to Sink B/1
  from Source B/1 -> Bin/1
  Cl/4 -> Cly/1
  Dl/7 -> DinSplit/5
  Dout/6 -> SE1x4/2
  Bin/6 -> from Source B/2
  BinSplit1/2 -> Brs/1
  Bin/5 -> Terminator16/1
  from Source D/1 -> Din/1
  Ain/1 -> Terminator1/1
  Cl/3 -> ClX/1
  AinSplit/1 -> Al/1
  DinSplit/3 -> Din/2
  BinSplit1/3 -> Bin/2
  Do/6 -> Subsystem/7(Do x)
  Subsystem/3(Co yk) -> Co/1
  Bout/3 -> BoutX/1
  Do/7 -> Subsystem/8(Do Kz)
  Brs/1 -> Terminator13/1
  Sink D/1 -> to Sink D/2
  Bl/5 -> Terminator47/1
  Cin/2 -> CinSplit/1
  Bo/6 -> Subsystem/1(Bo x)
  Al/5 -> Terminator40/1
  Co/2 -> SE1x3/1
  Bo/1 -> Terminator46/1
  Din/7 -> from Source D/3
  Ars/5 -> Terminator41/1
  Bo/3 -> BoX/1
  Sink A/2 -> to Sink A/3
  Brs/4 -> BrsY/1
  Bin/2 -> BinSplit1/1
  Ao/1 -> Terminator42/1
  Al/7 -> AinSplit/3
  to Sink A/1 -> sinks3/1(edge)
  Bin/1 -> Terminator10/1
  Ao2/2 -> SE1x7/1
  to Sink C/1 -> Cout3/1
  Drs/6 -> DinSplit/2
  Cl/5 -> Terminator38/1
  from Source A/2 -> sources4/1(edge)
  Ao2/4 -> AoY2/1
  Ari1/3 -> AriX1/1
  Co2/7 -> Subsystem1/17(Co Kz)
  Subsystem/4(Ao yk) -> Ao/1
  Ali1/4 -> AliY1/1
  CinSplit2/2 -> Cl2/1
  Brs/6 -> BinSplit1/4
  Ain2/2 -> AinSplit2/1
  SE1x7/1 -> Aout2/1
  Cout2/3 -> CoutX2/1
  Aout2/7 -> SE1x7/3
  Drs/7 -> DinSplit/3
  Ain2/3 -> AinX2/1
  Source A2/1 -> from Source A2/1
  Ao2/3 -> AoX2/1
  Do/1 -> Terminator45/1
  Cs1/6 -> CinSplit2/2
  Dout/7 -> SE1x4/3
  Ali1/6 -> AinSplit2/2
  Ao/6 -> Subsystem/21(Ao x)
  Aout/5 -> Terminator5/1
  to Sink A2/2 -> Aout2/2
  CinSplit/1 -> Crs/1
  Rk/1 -> Tzs1/1  "Rk"
  from Source B2/1 -> Brs2/1
  Brs2/3 -> BrsX2/1
  Brs2/4 -> BrsY2/1
  Bo2/3 -> BoX2/1
  Cs1/7 -> CinSplit2/3
  Cout2/4 -> CoutY2/1
  Cs1/4 -> CsY1/1
  Sink C2/2 -> to Sink C2/3
  Cout/2 -> to Sink C/1
  CinSplit2/3 -> Cin2/2
  Dout/2 -> to Sink D/1
  AinSplit2/1 -> Ali1/1
  Brs2/7 -> from Source B2/3
  Cl2/7 -> CinSplit2/5
  Cl2/6 -> CinSplit2/4
  Bl/6 -> BinSplit1/2
  Sink C2/1 -> to Sink C2/2
  Bin/4 -> BinY/1
  CinSplit2/1 -> Cs1/1
  AinSplit2/2 -> Ari1/1
  Source C2/1 -> from Source C2/1
  Bo2/2 -> to Sink B2/1
  Cin/4 -> CinY/1
  Bout/4 -> BoutY/1
  Subsystem1/3(Co yk) -> Co2/1
  Bo2/7 -> Subsystem1/2(Bo Kz)
  Ao/7 -> Subsystem/22(Ao Kz)
  AinSplit/3 -> Ain/2
  Aout2/2 -> to Sink A2/1
  Co2/4 -> CoY2/1
  Drs/4 -> DrsY/1
  Subsystem1/4(Ao yk) -> Ao2/1
  Dout/1 -> Terminator33/1
  Sink A2/1 -> to Sink A2/2
  Cin/5 -> Terminator25/1
  Cout2/6 -> SE1x8/2
  Cout2/7 -> SE1x8/3
  SE1x8/2 -> Co2/2
  Cin2/3 -> CinX2/1
  Bout/6 -> SE1x2/2
  Al/1 -> Terminator3/1
  Tz_dif/1 -> Tzs/3  "Tz_dif"
  SE1x8/1 -> Cout2/1
  Cin2/4 -> CinY2/1
  Ari1/7 -> AinSplit2/5
  SE1x7/2 -> Ao2/2
  CinSplit/2 -> Cl/1
  Ali1/7 -> AinSplit2/3
  from Source A2/1 -> Ain2/1
  AinSplit2/3 -> Ain2/2
  Ain2/6 -> from Source A2/2
  SE1x3/2 -> Co/2
  Drs/5 -> Terminator44/1
  from Source B3/2 -> Cout3/2
  Cout/1 -> Terminator24/1
  to Sink B2/1 -> Bo3/1
  Bo3/6 -> to Sink B2/2
  to Sink C2/2 -> Cout2/2
  Brs/7 -> BinSplit1/5
  Cin3/2 -> from Source C/1
  Brs3/6 -> to Sink B/2
  Brs3/7 -> to Sink B/3
  Ain2/7 -> from Source A2/3
  Cout3/6 -> to Sink C/2
  Subsystem/30(Bo yk) -> Bo/1
  Bo3/7 -> to Sink B2/3
  from Source C/2 -> Cin3/2
  Crs/3 -> CrsX/1
  Aout2/6 -> SE1x7/2
  Co2/2 -> SE1x8/1
  to Sink B/1 -> Brs3/1
  Brs2/6 -> from Source B2/2
  Sink A2/2 -> to Sink A2/3
  Ao2/6 -> Subsystem1/10(Ao x)
  Ari1/6 -> AinSplit2/4
  Bl/1 -> Terminator12/1
  Cin2/7 -> from Source C2/3
  from Source B2/2 -> Brs3/2
  Dout/5 -> Terminator32/1
  Ain2/4 -> AinY2/1
  Bo2/4 -> BoY2/1
  Cin2/6 -> from Source C2/2
  from Source C2/1 -> Cin2/1
  to Sink B2/2 -> Bo2/2
  SE1x4/1 -> Dout/1
  Cs1/3 -> CsX1/1
  Cout/6 -> SE1x3/2
  Ao2/7 -> Subsystem1/11(Ao Kz)
  Subsystem1/24(Bo yk) -> Bo2/1
  Cl2/4 -> ClY1/1
  Aout2/3 -> AoutX2/1
  Bo/5 -> Terminator11/1
  SE1x1/2 -> Ao/2
  Co2/3 -> CoX2/1
  Cin2/2 -> CinSplit2/1
  Bo2/6 -> Subsystem1/1(Bo x)
  Aout/1 -> Terminator6/1
  Ali1/3 -> AliX1/1
  Cout2/2 -> to Sink C2/1
  Din/3 -> DinX/1
  Cout3/7 -> to Sink C/3
  Ars/1 -> Terminator4/1
  Aout2/4 -> AoutY2/1
  from Source B/2 -> Bo3/2
  to Sink B/2 -> Bout/2
  Bo3/2 -> from Source B/1
  Kz_pre/1 -> Kzs/2  "Kz_pre"
  SE1x4/2 -> Do/2
  Cin3/6 -> to Sink B3/2
  Co2/6 -> Subsystem1/16(Co x)
  Cl2/3 -> ClX2/1
  to Sink B3/1 -> Cin3/1
  Subsystem/10(Al) -> Plus-Controller/3(Al)
  Subsystem/11(Ars) -> Plus-Controller/4(Ars)
  Subsystem/12(Bl) -> Plus-Controller/1(Bl)
  Subsystem/13(Brs) -> Plus-Controller/2(Brs)
  Subsystem/14(Cl) -> Plus-Controller/5(Cl)
  Subsystem/15(Crs) -> Plus-Controller/6(Crs)
  Subsystem/16(Dl) -> Plus-Controller/7(Dl)
  Subsystem/17(Drs) -> Plus-Controller/8(Drs)
  Subsystem/18(Al_Bo) -> Plus-Controller/9(Al_Bo)
  Subsystem/19(Ars_Do) -> Plus-Controller/10(Ars_Do)
  Subsystem/20(Ars_Co) -> Plus-Controller/11(Ars_Co)
  Subsystem/21(Bl_Do) -> Plus-Controller/12(Bl_Do)
  Subsystem/22(Brs_Co) -> Plus-Controller/13(Brs_Co)
  Subsystem/23(Brs_Ao) -> Plus-Controller/14(Brs_Ao)
  Subsystem/24(Cl_Ao) -> Plus-Controller/15(Cl_Ao)
  Subsystem/25(Crs_Bo) -> Plus-Controller/16(Crs_Bo)
  Subsystem/26(Crs_Do) -> Plus-Controller/17(Crs_Do)
  Subsystem/27(Dl_Co) -> Plus-Controller/18(Dl_Co)
  Subsystem/28(Drs_Ao) -> Plus-Controller/19(Drs_Ao)
  Subsystem/29(Drs_Bo) -> Plus-Controller/20(Drs_Bo)
  Plus-Controller/1(enAl) -> [CenAl], Subsystem/9(enAl)
  Plus-Controller/2(enAs) -> [CenAs], Subsystem/10(enAs)
  Plus-Controller/3(enAr) -> [CenAr], Subsystem/11(enAr)
  Plus-Controller/4(enBl) -> Subsystem/12(enBl), [CenBl]
  Plus-Controller/5(enBs) -> [CenBs], Subsystem/13(enBs)
  Plus-Controller/6(enBr) -> [CenBr], Subsystem/14(enBr)
  Plus-Controller/7(enCl) -> [CenCl], Subsystem/15(enCl)
  Plus-Controller/8(enCs) -> [CenCs], Subsystem/16(enCs)
  Plus-Controller/9(enCr) -> [CenCr], Subsystem/17(enCr)
  Plus-Controller/10(enDl) -> [CenDl], Subsystem/18(enDl)
  Plus-Controller/11(enDs) -> [CenDs], Subsystem/19(enDs)
  Plus-Controller/12(enDr) -> [CenDr], Subsystem/20(enDr)
  Cout4/4 -> CoutY3/1
  Controller for t-junction with lights/2 -> [RenCl], Subsystem3/8(Cl7)
  Controller for t-junction with lights/5 -> [RenBr], Subsystem3/5(Brs12)
  Ain3/3 -> AinX3/1
  Controller for t-junction with lights/3 -> [RenAr], Subsystem3/7(Ari4)
  Cl3/6 -> CinSplit3/4
  AinSplit3/2 -> Ari2/1
  Subsystem3/8(free_5) -> Controller for t-junction with lights/5
  Subsystem3/7(free_6) -> Controller for t-junction with lights/6
  Subsystem3/11(free_2) -> Controller for t-junction with lights/2
  Subsystem3/9(free_4) -> Controller for t-junction with lights/4
  Subsystem3/12(free_1) -> Controller for t-junction with lights/1
  Subsystem3/10(free_3) -> Controller for t-junction with lights/3
  SE1x10/2 -> Co3/2
  Controller for t-junction with lights/1 -> Subsystem3/9(Cs8), [RenCs]
  Bo4/3 -> BoX3/1
  Co3/7 -> Subsystem3/17(Co Kz)
  AinSplit3/1 -> Ali2/1
  AinSplit3/3 -> Ain3/2
  CinSplit3/2 -> Cl3/1
  Bo4/4 -> BoY3/1
  Ain3/7 -> from Source A3/3
  Subsystem3/4(Ao yk) -> Ao3/1
  Controller for t-junction with lights/4 -> [RenAl], Subsystem3/6(Ali3)
  CinSplit3/3 -> Cin4/2
  Cs2/3 -> CsX2/1
  Co3/2 -> SE1x10/1
  Aout3/7 -> SE1x9/3
  from Source B3/1 -> Brs4/1
  from Source A3/1 -> Ain3/1
  Ari2/3 -> AriX2/1
  Ali2/3 -> AliX2/1
  Cl3/3 -> ClX3/1
  Ao3/4 -> AoY3/1
  Co3/4 -> CoY3/1
  Ari2/4 -> AriY2/1
  Aout3/6 -> SE1x9/2
  Aout3/3 -> AoutX3/1
  Cs2/4 -> CsY2/1
  CinSplit3/1 -> Cs2/1
  Brs4/3 -> BrsX3/1
  Co3/3 -> CoX3/1
  Cs2/6 -> CinSplit3/2
  Ain3/4 -> AinY3/1
  Cl3/4 -> ClY2/1
  Cin4/6 -> from Source C3/2
  Sink A3/2 -> to Sink A3/3
  Controller for t-junction with lights/6 -> [RenBs], Subsystem3/4(Brs11)
  Subsystem3/3(Co yk) -> Co3/1
  to Sink B3/2 -> Bo4/2
  Bo4/2 -> to Sink B3/1
  Cin4/3 -> CinX3/1
  Bo4/7 -> Subsystem3/2(Bo Kz)
  to Sink C3/2 -> Cout4/2
  Cout4/2 -> to Sink C3/1
  from Source C3/1 -> Cin4/1
  Brs4/6 -> from Source B3/2
  Brs4/7 -> from Source B3/3
  SE1x10/1 -> Cout4/1
  Cout4/6 -> SE1x10/2
  Cin4/2 -> CinSplit3/1
  Sink C/1 -> to Sink C3/2
  Cin4/7 -> from Source C3/3
  Ari2/7 -> AinSplit3/5
  Cl3/7 -> CinSplit3/5
  Sink A3/1 -> to Sink A3/2
  Subsystem3/24(Bo yk) -> Bo4/1
  Co3/6 -> Subsystem3/16(Co x)
  Cs2/7 -> CinSplit3/3
  Bo4/6 -> Subsystem3/1(Bo x)
  SE1x9/2 -> Ao3/2
  SE1x9/1 -> Aout3/1
  Ali2/7 -> AinSplit3/3
  Ain3/2 -> AinSplit3/1
  Ao3/2 -> SE1x9/1
  Aout3/2 -> to Sink A3/1
  Brs4/4 -> BrsY3/1
  Ain3/6 -> from Source A3/2
  Aout3/4 -> AoutY3/1
  Source A3/1 -> from Source A3/1
  Cout4/7 -> SE1x10/3
  Ari2/6 -> AinSplit3/4
  Ali2/6 -> AinSplit3/2
  Cout4/3 -> CoutX3/1
  to Sink A3/2 -> Aout3/2
  Source C/1 -> from Source C3/1
  Ao3/3 -> AoX3/1
  Cin4/4 -> CinY3/1
  Ao3/7 -> Subsystem3/11(Ao Kz)
  Sink C/2 -> to Sink C3/3
  Ali2/4 -> AliY2/1
  Ao3/6 -> Subsystem3/10(Ao x)
  Cin3/7 -> to Sink B3/3
  Controller for t-junction with lights1/2 -> [LenCl], Subsystem1/8(Cl7)
  Controller for t-junction with lights1/5 -> Subsystem1/5(Brs12), [LenBr]
  Controller for t-junction with lights1/3 -> [LenAr], Subsystem1/7(Ari4)
  Subsystem1/8(free_5) -> Controller for t-junction with lights1/5
  Subsystem1/7(free_6) -> Controller for t-junction with lights1/6
  Subsystem1/11(free_2) -> Controller for t-junction with lights1/2
  Subsystem1/9(free_4) -> Controller for t-junction with lights1/4
  Subsystem1/12(free_1) -> Controller for t-junction with lights1/1
  Subsystem1/10(free_3) -> Controller for t-junction with lights1/3
  Controller for t-junction with lights1/1 -> [LenCs], Subsystem1/9(Cs8)
  Controller for t-junction with lights1/4 -> [LenAl], Subsystem1/6(Ali3)
  Controller for t-junction with lights1/6 -> [LenBs], Subsystem1/4(Brs11)
  from Source C2/2 -> sources7/1
  to Sink C2/1 -> sinks6/1(edge)
  [LenAr] -> deadtimes13/3(edge_enablestate)
  [LenAl] -> deadtimes12/3(edge_enablestate)
  Ari1/2 -> deadtimes13/1(x0z), Subsystem1/13(Ari x0)
  Subsystem1/5(Ali yk) -> deadtimes12/2(edge), Ali1/2
  Ali1/2 -> deadtimes12/1(x0z), Subsystem1/12(Ali x0)
  Subsystem1/6(Ari yk) -> deadtimes13/2(edge), Ari1/2
  Subsystem1/25(Brs yk) -> deadtimes11/2(edge), Brs2/2
  [LenBr] -> Logical Operator1/2
  Logical Operator1/1 -> deadtimes11/3(edge_enablestate)
  [LenBs] -> Logical Operator1/1
  Brs2/2 -> deadtimes11/1(x0z), Subsystem1/3(Brs x0)
  [LenCs] -> deadtimes15/3(edge_enablestate)
  [LenCl] -> deadtimes14/3(edge_enablestate)
  Cl2/2 -> deadtimes14/1(x0z), Subsystem1/15(Cl x0)
  Subsystem1/1(Cs yk) -> deadtimes15/2(edge), Cs1/2
  Cs1/2 -> deadtimes15/1(x0z), Subsystem1/14(Cs x0)
  Subsystem1/2(Cl yk) -> deadtimes14/2(edge), Cl2/2
  from Source A2/2 -> sources6/1(edge)
  to Sink A2/1 -> sinks5/1(edge)
  Logical Operator5/1 -> deadtimes17/3(edge_enablestate)
  Subsystem/7(Drs yk) -> deadtimes17/2(edge), Drs/2
  Subsystem/8(Dl yk) -> Dl/2, deadtimes16/2(edge)
  [CenDl] -> deadtimes16/3(edge_enablestate)
  [CenDr] -> Logical Operator5/2
  Drs/2 -> deadtimes17/1(x0z), Subsystem/5(Drs x0)
  Dl/2 -> deadtimes16/1(x0z), Subsystem/6(Dl x0)
  [CenDs] -> Logical Operator5/1
  [CenAs] -> Logical Operator3/1
  [CenAr] -> Logical Operator3/2
  [CenAl] -> deadtimes5/3(edge_enablestate)
  Al/2 -> deadtimes5/1(x0z), Subsystem/23(Al x0)
  Ars/2 -> deadtimes6/1(x0z), Subsystem/24(Ars x)
  Subsystem/5(Al yk) -> deadtimes5/2(edge), Al/2
  Subsystem/6(Ars yk) -> deadtimes6/2(edge), Ars/2
  Logical Operator3/1 -> deadtimes6/3(edge_enablestate)
  [CenBl] -> deadtimes9/3(edge_enablestate)
  Subsystem/31(Bl yk) -> Bl/2, deadtimes9/2(edge)
  Brs/2 -> deadtimes10/1(x0z), Subsystem/4(Brs x0)
  Logical Operator4/1 -> deadtimes10/3(edge_enablestate)
  [CenBr] -> Logical Operator4/2
  Subsystem/32(Brs yk) -> deadtimes10/2(edge), Brs/2
  [CenBs] -> Logical Operator4/1
  Bl/2 -> deadtimes9/1(x0z), Subsystem/3(Bl x0)
  [CenCr] -> Logical Operator2/2
  Crs/2 -> deadtimes8/1(x0z), Subsystem/25(Crs x0)
  [CenCs] -> Logical Operator2/1
  Subsystem/2(Cl yk) -> deadtimes7/2(edge), Cl/2
  Cl/2 -> deadtimes7/1(x0z), Subsystem/26(Cl x0)
  Subsystem/1(Crs yk) -> Crs/2, deadtimes8/2(edge)
  [CenCl] -> deadtimes7/3(edge_enablestate)
  Logical Operator2/1 -> deadtimes8/3(edge_enablestate)
  Cs2/2 -> deadtimes1/1(x0z), Subsystem3/14(Cs x0)
  [RenCl] -> deadtimes/3(edge_enablestate)
  Subsystem3/1(Cs yk) -> deadtimes1/2(edge), Cs2/2
  [RenCs] -> deadtimes1/3(edge_enablestate)
  Cl3/2 -> deadtimes/1(x0z), Subsystem3/15(Cl x0)
  Subsystem3/2(Cl yk) -> deadtimes/2(edge), Cl3/2
  Logical Operator/1 -> deadtimes4/3(edge_enablestate)
  [RenBr] -> Logical Operator/1
  Subsystem3/25(Brs yk) -> deadtimes4/2(edge), Brs4/2
  [RenBs] -> Logical Operator/2
  Brs4/2 -> Subsystem3/3(Brs x0), deadtimes4/1(x0z)
  Ari2/2 -> Subsystem3/13(Ari x0), deadtimes3/1(x0z)
  Subsystem3/5(Ali yk) -> Ali2/2, deadtimes2/2(edge)
  [RenAl] -> deadtimes2/3(edge_enablestate)
  [RenAr] -> deadtimes3/3(edge_enablestate)
  Subsystem3/6(Ari yk) -> deadtimes3/2(edge), Ari2/2
  Ali2/2 -> Subsystem3/12(Ali x0), deadtimes2/1(x0z)
  to Sink A3/1 -> sinks2/1(edge)
  from Source A3/2 -> sources2/1(edge)
  to Sink C3/1 -> sinks1/1(edge)
  from Source C3/2 -> sources1/1(edge)
  [CenCs] -> Scope/8
  [CenDr] -> Scope/12
  Plus-Controller/13(time) -> Scope/13
  [CenDs] -> Scope/11
  [CenCr] -> Scope/9
  [CenBr] -> Scope/6
  [CenAl] -> Scope/1
  [CenCl] -> Scope/7
  [CenDl] -> Scope/10
  [CenAs] -> Scope/2
  [CenAr] -> Scope/3
  [CenBl] -> Scope/4
  [CenBs] -> Scope/5

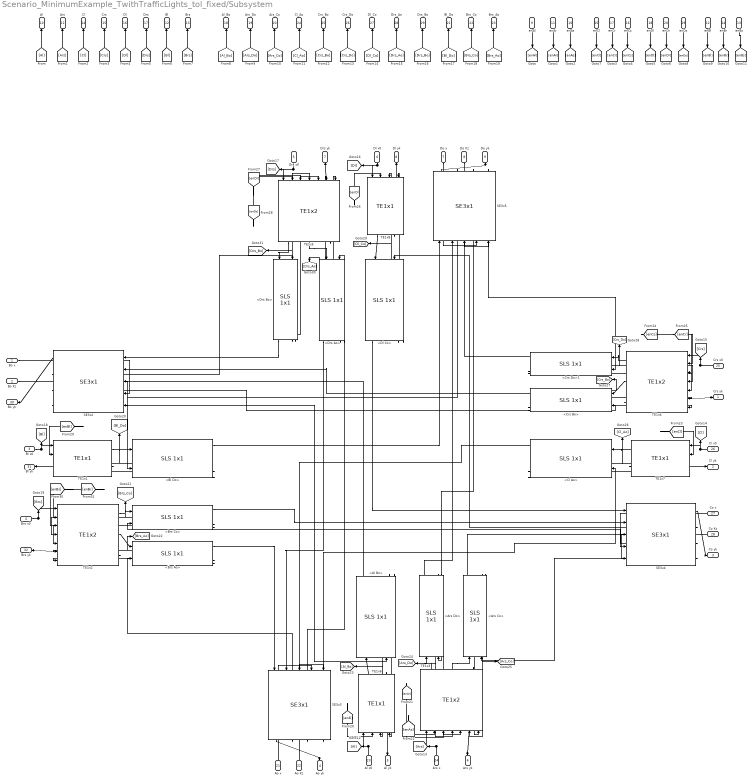
== system Scenario_MinimumExample_TwithTrafficLights_tol_fixed/Subsystem ==
  Bo x : Inport
  Bo Kz : Inport  Port=2
  Bl x0 : Inport  Port=3
  Brs x0 : Inport  Port=4
  Drs x0 : Inport  Port=5
  Dl x0 : Inport  Port=6
  Do x : Inport  Port=7
  Do Kz : Inport  Port=8
  enAl : Inport  Port=9
  enAs : Inport  Port=10
  enAr : Inport  Port=11
  enBl : Inport  Port=12
  enBs : Inport  Port=13
  enBr : Inport  Port=14
  enCl : Inport  Port=15
  enCs : Inport  Port=16
  enCr : Inport  Port=17
  enDl : Inport  Port=18
  enDs : Inport  Port=19
  enDr : Inport  Port=20
  Ao x : Inport  Port=21
  Ao Kz : Inport  Port=22
  Al x0 : Inport  Port=23
  Ars x : Inport  Port=24
  Crs x0 : Inport  Port=25
  Cl x0 : Inport  Port=26
  Co x : Inport  Port=27
  Co Kz : Inport  Port=28
  <Al Bo> : StreetLanesLibrary/SLS 1x1  Kz=Kz_left  Tz=Tz_left
  <Ars Co> : StreetLanesLibrary/SLS 1x1  Kz=Kz_right  Tz=Tz_right
  <Ars Do> : StreetLanesLibrary/SLS 1x1  Kz=Kz_straight  Tz=Tz_straight
  <Bl Do> : StreetLanesLibrary/SLS 1x1  Kz=Kz_left  Tz=Tz_left
  <Brs Ao> : StreetLanesLibrary/SLS 1x1  Kz=Kz_right  Tz=Tz_right
  <Brs Co> : StreetLanesLibrary/SLS 1x1  Kz=Kz_straight  Tz=Tz_straight
  <Cl Ao> : StreetLanesLibrary/SLS 1x1  Kz=Kz_left  Tz=Tz_left
  <Crs Bo> : StreetLanesLibrary/SLS 1x1  Kz=Kz_straight  Tz=Tz_straight
  <Crs Do>1 : StreetLanesLibrary/SLS 1x1  Kz=Kz_right  Tz=Tz_right
  <Dl Co> : StreetLanesLibrary/SLS 1x1  Kz=Kz_left  Tz=Tz_left
  <Drs Ao> : StreetLanesLibrary/SLS 1x1  Kz=Kz_straight  Tz=Tz_straight
  <Drs Bo> : StreetLanesLibrary/SLS 1x1  Kz=Kz_right  Tz=Tz_right
  SE3x{2..5} (4 alike) : EdgesLibrary/SE3x1  Rk1=Rk  Rk2=Rk  Rk3=Rk
  TE1x{1,6..8} (4 alike) : EdgesLibrary/TE1x1  Rk=Rk  slope=2000
  TE1x{2..5} (4 alike) : EdgesLibrary/TE1x2  Rk1=0.5*Rk  Rk2=0.5*Rk
  Crs yk : Outport
  Cl yk : Outport  Port=2
  Co yk : Outport  Port=3
  Ao yk : Outport  Port=4
  Al yk : Outport  Port=5
  Ars yk : Outport  Port=6
  Drs yk : Outport  Port=7
  Dl yk : Outport  Port=8
  Do yk : Outport  Port=9
  Al : Outport  Port=10
  Ars : Outport  Port=11
  Bl : Outport  Port=12
  Brs : Outport  Port=13
  Cl : Outport  Port=14
  Crs : Outport  Port=15
  Dl : Outport  Port=16
  Drs : Outport  Port=17
  Al_Bo : Outport  Port=18
  Ars_Do : Outport  Port=19
  Ars_Co : Outport  Port=20
  Bl_Do : Outport  Port=21
  Brs_Co : Outport  Port=22
  Brs_Ao : Outport  Port=23
  Cl_Ao : Outport  Port=24
  Crs_Bo : Outport  Port=25
  Crs_Do : Outport  Port=26
  Dl_Co : Outport  Port=27
  Drs_Ao : Outport  Port=28
  Drs_Bo : Outport  Port=29
  Bo yk : Outport  Port=30
  Bl yk : Outport  Port=31
  Brs yk : Outport  Port=32
  wires:
  SE3x2/1 -> Bo yk/1
  Bo Kz/1 -> SE3x2/5
  Bo x/1 -> SE3x2/4
  Bl x0/1 -> [Bl], TE1x1/1
  TE1x1/2 -> Bl yk/1
  Brs x0/1 -> [Brs], TE1x2/1
  TE1x2/3 -> Brs yk/1
  Ao x/1 -> SE3x3/4
  Ao Kz/1 -> SE3x3/5
  SE3x3/1 -> Ao yk/1
  Ars x/1 -> [Ars], TE1x3/1
  TE1x3/3 -> Ars yk/1
  Co Kz/1 -> SE3x4/5
  Co x/1 -> SE3x4/4
  SE3x4/1 -> Co yk/1
  TE1x4/3 -> Crs yk/1
  Crs x0/1 -> [Crs], TE1x4/1
  Do x/1 -> SE3x5/4
  Do Kz/1 -> SE3x5/5
  SE3x5/1 -> Do yk/1
  TE1x5/3 -> Drs yk/1
  Drs x0/1 -> [Drs], TE1x5/1
  TE1x4/2 -> <Crs Bo>/1
  <Crs Bo>/8 -> TE1x4/7
  <Crs Bo>/7 -> [Crs_Bo], TE1x4/6
  TE1x3/1 -> <Ars Do>/1
  <Ars Do>/8 -> TE1x3/5
  <Ars Do>/7 -> [Ars_Do], TE1x3/4
  TE1x2/1 -> <Brs Co>/1
  <Brs Co>/8 -> TE1x2/5
  <Brs Co>/7 -> [Brs_Co], TE1x2/4
  TE1x2/2 -> <Brs Ao>/1
  <Brs Ao>/8 -> TE1x2/7
  <Brs Ao>/7 -> TE1x2/6, [Brs_Ao]
  TE1x4/1 -> <Crs Do>1/1
  <Crs Do>1/8 -> TE1x4/5
  <Crs Do>1/7 -> [Crs_Do], TE1x4/4
  TE1x5/1 -> <Drs Bo>/1
  <Drs Bo>/8 -> TE1x5/5
  TE1x5/2 -> <Drs Ao>/1
  <Drs Ao>/8 -> TE1x5/7
  <Drs Ao>/7 -> [Drs_Ao], TE1x5/6
  TE1x3/2 -> <Ars Co>/1
  <Ars Co>/8 -> TE1x3/7
  TE1x1/1 -> <Bl Do>/1
  <Bl Do>/8 -> TE1x1/4
  <Bl Do>/7 -> [Bl_Do], TE1x1/3
  <Cl Ao>/7 -> TE1x7/3, [Cl_Ao]
  <Cl Ao>/8 -> TE1x7/4
  TE1x7/1 -> <Cl Ao>/1
  TE1x8/1 -> <Dl Co>/1
  <Dl Co>/8 -> TE1x8/4
  <Dl Co>/7 -> [Dl_Co], TE1x8/3
  TE1x6/1 -> <Al Bo>/1
  <Al Bo>/8 -> TE1x6/4
  <Al Bo>/7 -> TE1x6/3, [Al_Bo]
  <Drs Bo>/2 -> SE3x2/1
  SE3x2/2 -> <Drs Bo>/2
  <Crs Bo>/2 -> SE3x2/2
  SE3x2/3 -> <Crs Bo>/2
  <Al Bo>/2 -> SE3x2/3
  SE3x2/4 -> <Al Bo>/2
  <Crs Do>1/2 -> SE3x5/3
  SE3x5/4 -> <Crs Do>1/2
  SE3x5/3 -> <Ars Do>/2
  <Ars Do>/2 -> SE3x5/2
  <Bl Do>/2 -> SE3x5/1
  SE3x5/2 -> <Bl Do>/2
  SE3x4/4 -> <Ars Co>/2
  <Ars Co>/2 -> SE3x4/3
  SE3x4/3 -> <Brs Co>/2
  <Brs Co>/2 -> SE3x4/2
  SE3x4/2 -> <Dl Co>/2
  <Dl Co>/2 -> SE3x4/1
  SE3x3/2 -> <Brs Ao>/2
  <Brs Ao>/2 -> SE3x3/1
  SE3x3/3 -> <Drs Ao>/2
  <Drs Ao>/2 -> SE3x3/2
  SE3x3/4 -> <Cl Ao>/2
  <Cl Ao>/2 -> SE3x3/3
  <Ars Co>/7 -> TE1x3/6, [Ars_Co]
  Al x0/1 -> [Al], TE1x6/1
  TE1x6/2 -> Al yk/1
  Cl x0/1 -> [Cl], TE1x7/1
  TE1x7/2 -> Cl yk/1
  Dl x0/1 -> [Dl], TE1x8/1
  TE1x8/2 -> Dl yk/1
  [enAl] -> TE1x6/2
  [enAr] -> TE1x3/3
  [enAs] -> TE1x3/2
  [enCl] -> TE1x7/2
  [enCs] -> TE1x4/3
  [enCr] -> TE1x4/2
  [enDl] -> TE1x8/2
  [enBl] -> TE1x1/2
  [enBs] -> TE1x2/2
  [enBr] -> TE1x2/3
  [enDr] -> TE1x5/2
  [enDs] -> TE1x5/3
  <Drs Bo>/7 -> TE1x5/4, [Drs_Bo]
  [Al] -> Al/1
  [Ars] -> Ars/1
  [Cl] -> Cl/1
  [Crs] -> Crs/1
  [Dl] -> Dl/1
  [Drs] -> Drs/1
  [Bl] -> Bl/1
  [Brs] -> Brs/1
  [Al_Bo] -> Al_Bo/1
  [Ars_Do] -> Ars_Do/1
  [Ars_Co] -> Ars_Co/1
  [Cl_Ao] -> Cl_Ao/1
  [Crs_Bo] -> Crs_Bo/1
  [Crs_Do] -> Crs_Do/1
  [Dl_Co] -> Dl_Co/1
  [Drs_Ao] -> Drs_Ao/1
  [Drs_Bo] -> Drs_Bo/1
  [Bl_Do] -> Bl_Do/1
  [Brs_Co] -> Brs_Co/1
  [Brs_Ao] -> Brs_Ao/1
  enAl/1 -> [enAl]
  enAr/1 -> [enAr]
  enAs/1 -> [enAs]
  enCl/1 -> [enCl]
  enCr/1 -> [enCr]
  enCs/1 -> [enCs]
  enDl/1 -> [enDl]
  enDr/1 -> [enDr]
  enDs/1 -> [enDs]
  enBl/1 -> [enBl]
  enBr/1 -> [enBr]
  enBs/1 -> [enBs]
